simulink library "EmE_MBD_Blockset"  (R2018a)
settings: Solver=ode1  StartTime=0.0  StopTime=Inf  FixedStep=0.001  RelTol=1e-3  EnableMultiTasking=on
PostLoadFcn:
  | , if any(exist('dsrtsu_mdlpostloadfcn', 'file') == [2, 3, 6]), try dsrtsu_mdlpostloadfcn('Execute', bdroot); catch fprintf('Error in PostLoadFcn (dsrtsu_mdlpostloadfcn) for model "%s":\n %s\n', bdroot, lasterr); end, end,
undefined symbols (not defined in the file or in its folder): ENUM_TSC1_CONTROL_PURPOSE_T, gcbh, GLB_SWITCH_T
libraries: simulink x237, $bdroot x115, simulink_need_slupdate x26, MotoHawk_lib x13, simulink_extras x3
(part 5 of 11)

== system EmE_MBD_Blockset/Discrete/PT1_First_order_lag/Cubic_Approximation ==
  In1 : Inport
  Add2 : Sum  Inputs=++++  InputSameDT=on
  Constant2 : Constant
  Product{4..8} (5 alike) : Product  InputSameDT=on
  cubic_appr_x2_factor : Constant  Value=0.468222
  cubic_appr_x3_factor : Constant  Value=0.105562
  cubic_appr_x_factor : Constant  Value=0.995043
  Out1 : Outport
  wires:
  Product4/1 -> Product7/1, Product5/1
  cubic_appr_x_factor/1 -> Product6/2
  Product8/1 -> Add2/4
  cubic_appr_x3_factor/1 -> Product8/2
  Product5/1 -> Product8/1
  cubic_appr_x2_factor/1 -> Product7/2
  Product6/1 -> Add2/2
  Add2/1 -> Out1/1
  Product7/1 -> Add2/3
  Constant2/1 -> Add2/1
  In1/1 -> Product4/1, Product4/2, Product5/2, Product6/1

== system EmE_MBD_Blockset/Discrete/Turn_off_delay/SR flip-flop1 ==
  Sp : Inport
  R : Inport  Port=2
  Logical Operator : Logic  OutDataTypeStr=boolean
  Logical Operator1 : Logic  Operator=OR  OutDataTypeStr=boolean
  Logical Operator2 : Logic  Operator=NOT  OutDataTypeStr=boolean
  Logical Operator3 : Logic  Operator=NOT  OutDataTypeStr=boolean
  Unit_Delay : UnitDelay  InitialCondition=false  SampleTime=-1
      settings: AttributesFormatString=IC: %<vinit>
  Q : Outport
  !Q : Outport  Port=2
  wires:
  Logical Operator2/1 -> !Q/1
  Sp/1 -> Logical Operator1/1
  Logical Operator1/1 -> Q/1, Unit_Delay/1, Logical Operator2/1
  Logical Operator/1 -> Logical Operator1/2
  Logical Operator3/1 -> Logical Operator/1
  Unit_Delay/1 -> Logical Operator/2
  R/1 -> Logical Operator3/1

== system EmE_MBD_Blockset/Logic and Bit Operations/D flip-flop with SR/Enabled and Triggered Subsystem ==
  In1 : Inport  LatchByDelayingOutsideSignal=on
  Enable : EnablePort
  Trigger : TriggerPort  VariantControl=(inherit)  StatesWhenEnabling=reset
  Logical Operator : Logic  Operator=NOT  OutDataTypeStr=boolean
  Out1 : Outport  OutputWhenDisabled=reset  InitialOutput=false
  Out2 : Outport  Port=2  OutputWhenDisabled=reset  InitialOutput=true
  wires:
  In1/1 -> Logical Operator/1, Out1/1
  Logical Operator/1 -> Out2/1

== system EmE_MBD_Blockset/User-Defined Functions/Snoop/CCP_ETC_SS1 ==
  note: Define Signal information for desired signals
  note: Calculate and Track
      | current PID and Offset
  note: Detect if the new CCP command is
      | new and one of interest.
  note: Continuously decode all
      | CCP commands
  note: Form the message pairing
      | only after recieving a
      | WRITE_DAQ message
      | command
  function : TriggerPort  TriggerType=function-call  VariantControl=(inherit)
  Bus Selector : BusSelector  OutputSignals=ODT_Number,DAQ_Number
  Bus Selector1 : BusSelector  OutputSignals=Element_Size,Memory_Address
  CCP Signal Data Configuration : Subsystem
  Calculate Data Location : Subsystem
  Process CCP Commands : Subsystem
  Read CAN Raw1 : MotoHawk_lib/CAN Blocks/Read CAN Raw  nam='CAN_2'  bus=-2  id_ext=1  id=hex2dec('EF00F8')  id_mask=hex2dec('1fffffff')  pay=[]  pay_mask=[]  queue=20  slot='CCP_ATI'  valid=off  stale=on
      settings: SourceProductName=MotoHawk
  Recieve Count : Subsystem
      mask Display: disp('RCV COUNT')
  Signal Data Pairing : Subsystem
  Terminator{,1..3,5} (5 alike) : Terminator
  Update Detect : Subsystem
  DAQ_Info : Outport
  wires:
  Process CCP Commands/6(STRT_STP) -> Signal Data Pairing/5(STRT_STP)
  Bus Selector/2 -> Calculate Data Location/5(DAQ_Number)  "<DAQ_Number>"
  Read CAN Raw1/5 -> Process CCP Commands/1(CCP_Raw)
  Signal Data Pairing/1(DAQ_Info) -> DAQ_Info/1
  CCP Signal Data Configuration/1(CCP_Signal_Info) -> Signal Data Pairing/6(Signal_Info)
  Calculate Data Location/2(Offset) -> Signal Data Pairing/3(Offset)
  Calculate Data Location/1(PID) -> Signal Data Pairing/2(PID)
  Update Detect/2(Set_Update) -> Calculate Data Location/2(Set_Update)
  Update Detect/1(Write_Update) -> Signal Data Pairing/1(Write_Update), Calculate Data Location/1(Write_Update)
  Bus Selector1/1 -> Calculate Data Location/6(Element_Size)  "<Element_Size>"
  Bus Selector/1 -> Calculate Data Location/4(ODT_Number)  "<ODT_Number>"
  Process CCP Commands/3(GET) -> Terminator/1
  Bus Selector1/2 -> Signal Data Pairing/4(Memory_Address)  "<Memory_Address>"
  Process CCP Commands/5(WRITE) -> Bus Selector1/1
  Process CCP Commands/4(SET) -> Bus Selector/1
  Process CCP Commands/2(Newest_Cmd) -> Update Detect/2(Newest_Cmd), Calculate Data Location/3(Newest_CMD)
  Process CCP Commands/1(CTR) -> Update Detect/1(CTR)
  Read CAN Raw1/1 -> Terminator2/1
  Read CAN Raw1/4 -> Terminator1/1
  Read CAN Raw1/3 -> Terminator5/1
  Read CAN Raw1/2 -> Terminator3/1

== system EmE_MBD_Blockset/User-Defined Functions/Snoop/CCP_ETC_SS2 ==
  DAQ_Info : Inport
  function : TriggerPort  TriggerType=function-call  VariantControl=(inherit)
  CCP_Parameter_Decode : Subsystem
  Read CAN Raw : MotoHawk_lib/CAN Blocks/Read CAN Raw  nam='CAN_2'  bus=-2  id_ext=1  id=hex2dec('1CEFF800')  id_mask=hex2dec('1fffffff')  pay=[]  pay_mask=[]  queue=10  slot='CCP_ETC'  valid=off  stale=off
      settings: SourceProductName=MotoHawk
  Recieve Count : Subsystem
      mask Display: disp('RCV COUNT')
  Terminator1 : Terminator
  Terminator2 : Terminator
  Terminator4 : Terminator
  RCV_DATA : Outport
  wires:
  DAQ_Info/1 -> CCP_Parameter_Decode/1(DAQ_Info)
  Read CAN Raw/4 -> CCP_Parameter_Decode/2(Data)
  CCP_Parameter_Decode/1(CCP_Parameters) -> RCV_DATA/1
  Read CAN Raw/3 -> Terminator2/1
  Read CAN Raw/2 -> Terminator1/1
  Read CAN Raw/1 -> Terminator4/1

== system EmE_MBD_Blockset/User-Defined Functions/Snoop/Defaulting ==
  RCV_DATA : Inport
  DAQ_Info : Inport  Port=2
  function : TriggerPort  TriggerType=function-call  VariantControl=(inherit)
  Bus Creator : BusCreator  Inputs=24
  Bus Creator1 : BusCreator  Inputs=2
  Bus Selector3 : BusSelector  OutputSignals=Data.Signal1,Info.Signal_Def1.F_Defined,Data.Signal2,Info.Signal_Def2.F_Defined,Data.Signal3,Info.Signal_Def3.F_Defined,Data.Signal4,Info.Signal_Def4.F_Defined,Data.Signal5,Info.Signal_Def5.F_Defined,Data.Signal6,Info.Signal_Def6.F_Defined,Data.Signal7,Info.Signal_Def7.F_Defined,Data.Signal8,Info.Signal_Def8.F_Defined,Data.Signal9,Info.Signal_Def9.F_Defined,Data.Signal10,Info.Signal_Def10.F_Defined,Data.Signal11,Info.Signal_Def11.F_Defined,Data.Signal12,Info.Signal_Def12.F_Defined
  DEFAULT1 : Subsystem  mask{Parameter1=12}
      mask prompts: Parameter1 "CCP_SIG_DEFAULT"
      mask Display: disp(get(gcbh,'name'))
  DEFAULT10 : Subsystem  mask{Parameter1=12}
      mask prompts: Parameter1 "CCP_SIG_DEFAULT"
      mask Display: disp(get(gcbh,'name'))
  DEFAULT11 : Subsystem  mask{Parameter1=12}
      mask prompts: Parameter1 "CCP_SIG_DEFAULT"
      mask Display: disp(get(gcbh,'name'))
  DEFAULT12 : Subsystem  mask{Parameter1=12}
      mask prompts: Parameter1 "CCP_SIG_DEFAULT"
      mask Display: disp(get(gcbh,'name'))
  DEFAULT2 : Subsystem  mask{Parameter1=12}
      mask prompts: Parameter1 "CCP_SIG_DEFAULT"
      mask Display: disp(get(gcbh,'name'))
  DEFAULT3 : Subsystem  mask{Parameter1=12}
      mask prompts: Parameter1 "CCP_SIG_DEFAULT"
      mask Display: disp(get(gcbh,'name'))
  DEFAULT4 : Subsystem  mask{Parameter1=12}
      mask prompts: Parameter1 "CCP_SIG_DEFAULT"
      mask Display: disp(get(gcbh,'name'))
  DEFAULT5 : Subsystem  mask{Parameter1=12}
      mask prompts: Parameter1 "CCP_SIG_DEFAULT"
      mask Display: disp(get(gcbh,'name'))
  DEFAULT6 : Subsystem  mask{Parameter1=12}
      mask prompts: Parameter1 "CCP_SIG_DEFAULT"
      mask Display: disp(get(gcbh,'name'))
  DEFAULT7 : Subsystem  mask{Parameter1=12}
      mask prompts: Parameter1 "CCP_SIG_DEFAULT"
      mask Display: disp(get(gcbh,'name'))
  DEFAULT8 : Subsystem  mask{Parameter1=12}
      mask prompts: Parameter1 "CCP_SIG_DEFAULT"
      mask Display: disp(get(gcbh,'name'))
  DEFAULT9 : Subsystem  mask{Parameter1=12}
      mask prompts: Parameter1 "CCP_SIG_DEFAULT"
      mask Display: disp(get(gcbh,'name'))
  Recieve Count : Subsystem
      mask Display: disp('DFLT COUNT')
  motohawk_calibration2 : MotoHawk_lib/Calibration & Probing Blocks/motohawk_calibration  nam='CCP_SNOOP_RESET_DELAY'  val=100  storage=Calibration  show_more=on  name_source=Use Parameter  data_type=Inherit via back propagation  read_level=1  write_level=1  ovr_cals=on  view_as=Number  enum_struct={'Disabled', 'Enabled'}  vector_style=Wide Row  use_help_units=off  help=''  units=''  use_header_enum=off  row_header_enum={}  col_header_enum={}  use_min_max=off  min_val=-inf  max_val=inf  use_precision=off  precision=''  gain=1  offset=0  exp=1  use_mototune_group=on  mototune_group='CCP_Snoop'  data_stores=motohawk_sfun_calibration_data_stores
      settings: SourceProductName=MotoHawk
  CCP_ETC_Data : Outport
  wires:
  motohawk_calibration2/1 -> DEFAULT2/2(reset_delay), DEFAULT3/2(reset_delay), DEFAULT4/2(reset_delay), DEFAULT5/2(reset_delay), DEFAULT6/2(reset_delay), DEFAULT7/2(reset_delay), DEFAULT8/2(reset_delay), DEFAULT9/2(reset_delay), DEFAULT10/2(reset_delay), DEFAULT11/2(reset_delay), DEFAULT12/2(reset_delay), DEFAULT1/2(reset_delay)
  Bus Creator/1 -> CCP_ETC_Data/1
  DEFAULT12/2(F_Defined) -> Bus Creator/24  "CA_Vehicle_speed_defined"
  DEFAULT12/1(Signal) -> Bus Creator/23  "CA_Vehicle_speed"
  DEFAULT11/2(F_Defined) -> Bus Creator/22  "CPM_Crank_power_defined"
  DEFAULT11/1(Signal) -> Bus Creator/21  "CPM_Crank_power"
  DEFAULT10/2(F_Defined) -> Bus Creator/20  "Air_temp_post_int_Value_defined"
  DEFAULT10/1(Signal) -> Bus Creator/19  "Air_temp_post_int_Value"
  DEFAULT9/2(F_Defined) -> Bus Creator/18  "F_CPM_Int_enabled_defined"
  DEFAULT9/1(Signal) -> Bus Creator/17  "F_CPM_Int_enabled"
  DEFAULT8/2(F_Defined) -> Bus Creator/16  "CREC_Eng_run_time_since_key_on_defined"
  DEFAULT8/1(Signal) -> Bus Creator/15  "CREC_Eng_run_time_since_key_on"
  DEFAULT7/2(F_Defined) -> Bus Creator/14  "CA_Cool_temp_value_defined"
  DEFAULT7/1(Signal) -> Bus Creator/13  "CA_Cool_temp_value"
  DEFAULT6/2(F_Defined) -> Bus Creator/12  "CA_Engine_speed_defined"
  DEFAULT6/1(Signal) -> Bus Creator/11  "CA_Engine_speed"
  DEFAULT5/2(F_Defined) -> Bus Creator/10  "CA_Ambient_air_press_value_defined"
  DEFAULT5/1(Signal) -> Bus Creator/9  "CA_Ambient_air_press_value"
  DEFAULT4/2(F_Defined) -> Bus Creator/8  "AMF_Fresh_air_defined"
  DEFAULT4/1(Signal) -> Bus Creator/7  "AMF_Fresh_air"
  DEFAULT3/2(F_Defined) -> Bus Creator/6  "CPM_Air_temp_pre_int_defined"
  DEFAULT3/1(Signal) -> Bus Creator/5  "CPM_Air_temp_pre_int"
  DEFAULT2/2(F_Defined) -> Bus Creator/4  "CA_Ecfan_fspd_value_defined"
  DEFAULT2/1(Signal) -> Bus Creator/3  "CA_Ecfan_fspd_value"
  Bus Selector3/24 -> DEFAULT12/3(f_defined)  "<F_Defined>"
  Bus Selector3/23 -> DEFAULT12/1(signal)  "<Signal12>"
  Bus Selector3/22 -> DEFAULT11/3(f_defined)  "<F_Defined>"
  Bus Selector3/21 -> DEFAULT11/1(signal)  "<Signal11>"
  Bus Selector3/20 -> DEFAULT10/3(f_defined)  "<F_Defined>"
  Bus Selector3/19 -> DEFAULT10/1(signal)  "<Signal10>"
  Bus Selector3/18 -> DEFAULT9/3(f_defined)  "<F_Defined>"
  Bus Selector3/17 -> DEFAULT9/1(signal)  "<Signal9>"
  Bus Selector3/16 -> DEFAULT8/3(f_defined)  "<F_Defined>"
  Bus Selector3/15 -> DEFAULT8/1(signal)  "<Signal8>"
  Bus Selector3/14 -> DEFAULT7/3(f_defined)  "<F_Defined>"
  Bus Selector3/13 -> DEFAULT7/1(signal)  "<Signal7>"
  Bus Selector3/12 -> DEFAULT6/3(f_defined)  "<F_Defined>"
  Bus Selector3/11 -> DEFAULT6/1(signal)  "<Signal6>"
  Bus Selector3/10 -> DEFAULT5/3(f_defined)  "<F_Defined>"
  Bus Selector3/9 -> DEFAULT5/1(signal)  "<Signal5>"
  Bus Selector3/8 -> DEFAULT4/3(f_defined)  "<F_Defined>"
  Bus Selector3/7 -> DEFAULT4/1(signal)  "<Signal4>"
  Bus Selector3/6 -> DEFAULT3/3(f_defined)  "<F_Defined>"
  Bus Selector3/5 -> DEFAULT3/1(signal)  "<Signal3>"
  Bus Selector3/4 -> DEFAULT2/3(f_defined)  "<F_Defined>"
  Bus Selector3/3 -> DEFAULT2/1(signal)  "<Signal2>"
  Bus Selector3/2 -> DEFAULT1/3(f_defined)  "<F_Defined>"
  Bus Selector3/1 -> DEFAULT1/1(signal)  "<Signal1>"
  RCV_DATA/1 -> Bus Creator1/1  "Data"
  Bus Creator1/1 -> Bus Selector3/1
  DEFAULT1/2(F_Defined) -> Bus Creator/2  "CA_Ambient_air_temp_value_defined"
  DEFAULT1/1(Signal) -> Bus Creator/1  "CA_Ambient_air_temp_value"
  DAQ_Info/1 -> Bus Creator1/2  "Info"

== system EmE_MBD_Blockset/Controllers/Generic_PID_Governor_3/Calculate_PID_terms/Calculate_D_term ==
  GPID_Kd : Inport
  GPID_dT : Inport  Port=2
  F_GPID_reset_gov : Inport  Port=3
  GPID_control_error : Inport  Port=4
  GPID_T_filt_d : Inport  Port=5
  Enable : EnablePort  StatesWhenEnabling=reset
      settings: AttributesFormatString=States when enabling: %<StatesWhenEnabling>
  Divide : Product  Inputs=*/*  InputSameDT=on
  LPF_first_order : $bdroot/Discrete/LPF_first_order
  Subtract : Sum  Inputs=+-  InputSameDT=on
  Unit Delay Resettable External IC : simulink_need_slupdate/Unit Delay Resettable External IC  tsamp=-1
      settings: SourceProductName=Simulink  SourceProductBaseCode=SL
  GPID_d_term : Outport  OutputWhenDisabled=reset  InitialOutput=0
      settings: AttributesFormatString=IC: %<InitialOutput>\nDisabled value: %<OutputWhenDisabled>
  wires:
  GPID_control_error/1 -> LPF_first_order/2, LPF_first_order/3
  F_GPID_reset_gov/1 -> Unit Delay Resettable External IC/2, LPF_first_order/1
  GPID_dT/1 -> Divide/2, LPF_first_order/5
  GPID_T_filt_d/1 -> LPF_first_order/4
  LPF_first_order/1 -> Divide/1
  GPID_Kd/1 -> Divide/3
  Divide/1 -> Subtract/1, Unit Delay Resettable External IC/1, Unit Delay Resettable External IC/3
  Unit Delay Resettable External IC/1 -> Subtract/2
  Subtract/1 -> GPID_d_term/1

== system EmE_MBD_Blockset/Controllers/Generic_PID_Governor_3/Calculate_PID_terms/Calculate_I_term ==
  GPID_p_term : Inport
  GPID_Ki : Inport  Port=2
  GPID_actual_system_output : Inport  Port=3
  GPID_control_error : Inport  Port=4
  F_GPID_reset_gov : Inport  Port=5
  GPID_dT : Inport  Port=6
  GPID_feed_forward : Inport  Port=7
  F_GPID_aw_cond_integration : Inport  Port=8
  GPID_aw_hysteresis : Inport  Port=9
  F_GPID_aw_hold_i_term : Inport  Port=10
  GPID_output_unlim_prev : Inport  Port=11
  Enable : EnablePort  StatesWhenEnabling=reset
      settings: AttributesFormatString=States when enabling: %<StatesWhenEnabling>
  Calculate_integral_term : Subsystem
  Initialize_integral_term : Subsystem
  Prevent_integral_term_windup : Subsystem
  Unit_Delay : UnitDelay  SampleTime=-1
      settings: AttributesFormatString=IC: %<vinit>
  GPID_i_term : Outport  OutputWhenDisabled=reset  InitialOutput=0
      settings: AttributesFormatString=IC: %<InitialOutput>\nDisabled value: %<OutputWhenDisabled>
  F_GPID_hold_i_term : Outport  Port=2  OutputWhenDisabled=reset  InitialOutput=false
      settings: AttributesFormatString=IC: %<InitialOutput>\nDisabled value: %<OutputWhenDisabled>
  wires:
  Calculate_integral_term/1(GPID_i_term) -> GPID_i_term/1, Unit_Delay/1
  Initialize_integral_term/1(GPID_i_sum_error_init) -> Calculate_integral_term/3(GPID_i_sum_error_init)
  Prevent_integral_term_windup/1(F_GPID_hold_i_term) -> Calculate_integral_term/6(F_GPID_hold_i_term), F_GPID_hold_i_term/1
  GPID_dT/1 -> Initialize_integral_term/1(GPID_dT), Calculate_integral_term/1(GPID_dT)
  F_GPID_reset_gov/1 -> Prevent_integral_term_windup/4(F_GPID_reset_gov), Initialize_integral_term/Enable, Calculate_integral_term/2(F_GPID_reset_gov)
  GPID_feed_forward/1 -> Initialize_integral_term/2(GPID_feed_forward)
  GPID_Ki/1 -> Initialize_integral_term/6(GPID_Ki), Calculate_integral_term/5(GPID_Ki), Prevent_integral_term_windup/1(GPID_Ki)
  GPID_control_error/1 -> Initialize_integral_term/5(GPID_control_error), Calculate_integral_term/4(GPID_control_error), Prevent_integral_term_windup/2(GPID_control_error)
  GPID_actual_system_output/1 -> Initialize_integral_term/4(GPID_actual_system_output), Prevent_integral_term_windup/3(GPID_actual_system_output)
  GPID_p_term/1 -> Initialize_integral_term/3(GPID_p_term)
  GPID_output_unlim_prev/1 -> Prevent_integral_term_windup/5(GPID_output_unlim_prev)
  F_GPID_aw_cond_integration/1 -> Prevent_integral_term_windup/6(F_GPID_aw_cond_integration)
  GPID_aw_hysteresis/1 -> Prevent_integral_term_windup/7(GPID_aw_hysteresis)
  F_GPID_aw_hold_i_term/1 -> Prevent_integral_term_windup/8(F_GPID_aw_hold_i_term)
  Unit_Delay/1 -> Prevent_integral_term_windup/9(GPID_i_term_prev)

== system EmE_MBD_Blockset/Controllers/Generic_PID_Governor_3/Calculate_PID_terms/Calculate_P_term ==
  GPID_Kp : Inport
  GPID_control_error : Inport  Port=2
  Product : Product  InputSameDT=on
  GPID_p_term : Outport
  wires:
  Product/1 -> GPID_p_term/1
  GPID_control_error/1 -> Product/2
  GPID_Kp/1 -> Product/1

== system EmE_MBD_Blockset/Controllers/Generic_PID_Governor_4/Calculate_PID_terms/Calculate_D_term ==
  GPID_Kd : Inport
  GPID_dT : Inport  Port=2
  F_GPID_reset_gov : Inport  Port=3
  GPID_control_error : Inport  Port=4
  GPID_T_filt_d : Inport  Port=5
  Enable : EnablePort  StatesWhenEnabling=reset
      settings: AttributesFormatString=States when enabling: %<StatesWhenEnabling>
  Divide : Product  Inputs=*/*  InputSameDT=on
  LPF_first_order : $bdroot/Discrete/LPF_first_order
  Subtract : Sum  Inputs=+-  InputSameDT=on
  Unit Delay Resettable External IC : simulink_need_slupdate/Unit Delay Resettable External IC  tsamp=-1
      settings: SourceProductName=Simulink  SourceProductBaseCode=SL
  GPID_d_term : Outport  OutputWhenDisabled=reset  InitialOutput=0
      settings: AttributesFormatString=IC: %<InitialOutput>\nDisabled value: %<OutputWhenDisabled>
  wires:
  GPID_control_error/1 -> LPF_first_order/2, LPF_first_order/3
  F_GPID_reset_gov/1 -> Unit Delay Resettable External IC/2, LPF_first_order/1
  GPID_dT/1 -> Divide/2, LPF_first_order/5
  GPID_T_filt_d/1 -> LPF_first_order/4
  LPF_first_order/1 -> Divide/1
  GPID_Kd/1 -> Divide/3
  Divide/1 -> Subtract/1, Unit Delay Resettable External IC/1, Unit Delay Resettable External IC/3
  Unit Delay Resettable External IC/1 -> Subtract/2
  Subtract/1 -> GPID_d_term/1

== system EmE_MBD_Blockset/Controllers/Generic_PID_Governor_4/Calculate_PID_terms/Calculate_I_term ==
  GPID_p_term : Inport
  GPID_Ki : Inport  Port=2
  GPID_actual_system_output : Inport  Port=3
  GPID_control_error : Inport  Port=4
  F_GPID_reset_gov : Inport  Port=5
  GPID_dT : Inport  Port=6
  GPID_feed_forward : Inport  Port=7
  F_GPID_aw_cond_integration : Inport  Port=8
  GPID_aw_hysteresis : Inport  Port=9
  F_GPID_aw_hold_i_term : Inport  Port=10
  GPID_output_unlim_prev : Inport  Port=11
  GPID_output_delta : Inport  Port=12
  Enable : EnablePort  StatesWhenEnabling=reset
      settings: AttributesFormatString=States when enabling: %<StatesWhenEnabling>
  Calculate_integral_term : Subsystem
  Initialize_integral_term : Subsystem
  Prevent_integral_term_windup : Subsystem
  Unit_Delay : UnitDelay  SampleTime=-1
      settings: AttributesFormatString=IC: %<vinit>
  GPID_i_term : Outport  OutputWhenDisabled=reset  InitialOutput=0
      settings: AttributesFormatString=IC: %<InitialOutput>\nDisabled value: %<OutputWhenDisabled>
  F_GPID_hold_i_term : Outport  Port=2  OutputWhenDisabled=reset  InitialOutput=false
      settings: AttributesFormatString=IC: %<InitialOutput>\nDisabled value: %<OutputWhenDisabled>
  wires:
  Calculate_integral_term/1(GPID_i_term) -> GPID_i_term/1, Unit_Delay/1
  Initialize_integral_term/1(GPID_i_sum_error_init) -> Calculate_integral_term/3(GPID_i_sum_error_init)
  Prevent_integral_term_windup/1(F_GPID_hold_i_term) -> Calculate_integral_term/7(F_GPID_hold_i_term), F_GPID_hold_i_term/1
  GPID_dT/1 -> Initialize_integral_term/1(GPID_dT), Calculate_integral_term/1(GPID_dT)
  F_GPID_reset_gov/1 -> Prevent_integral_term_windup/4(F_GPID_reset_gov), Initialize_integral_term/Enable, Calculate_integral_term/2(F_GPID_reset_gov)
  GPID_feed_forward/1 -> Initialize_integral_term/2(GPID_feed_forward)
  GPID_Ki/1 -> Initialize_integral_term/6(GPID_Ki), Calculate_integral_term/5(GPID_Ki), Prevent_integral_term_windup/1(GPID_Ki)
  GPID_control_error/1 -> Initialize_integral_term/5(GPID_control_error), Calculate_integral_term/4(GPID_control_error), Prevent_integral_term_windup/2(GPID_control_error)
  GPID_actual_system_output/1 -> Initialize_integral_term/4(GPID_actual_system_output), Prevent_integral_term_windup/3(GPID_actual_system_output)
  GPID_p_term/1 -> Initialize_integral_term/3(GPID_p_term)
  GPID_output_unlim_prev/1 -> Prevent_integral_term_windup/5(GPID_output_unlim_prev)
  F_GPID_aw_cond_integration/1 -> Prevent_integral_term_windup/6(F_GPID_aw_cond_integration)
  GPID_aw_hysteresis/1 -> Prevent_integral_term_windup/7(GPID_aw_hysteresis)
  F_GPID_aw_hold_i_term/1 -> Prevent_integral_term_windup/8(F_GPID_aw_hold_i_term)
  Unit_Delay/1 -> Prevent_integral_term_windup/9(GPID_i_term_prev)
  GPID_output_delta/1 -> Calculate_integral_term/6(GPID_output_delta)

== system EmE_MBD_Blockset/Controllers/Generic_PID_Governor_4/Calculate_PID_terms/Calculate_P_term ==
  GPID_Kp : Inport
  GPID_control_error : Inport  Port=2
  Product : Product  InputSameDT=on
  GPID_p_term : Outport
  wires:
  Product/1 -> GPID_p_term/1
  GPID_control_error/1 -> Product/2
  GPID_Kp/1 -> Product/1

== system EmE_MBD_Blockset/User-Defined Functions/Snoop/CCP_ETC_SS1/CCP Signal Data Configuration ==
  note: Use Byte 1
      | 0 = Float
      | 1 = Use
  note: Use Byte 2
      | 0 = Don't Use
      | 1 = Use
  note: Use Byte 3-4
      | 0 = Don't Use
      | 1 = Use
  note: Signage
      | 0 = Unsigned
      | 1 = Signed
  note: Signal Types
      | 0001 = uchar     UBYTE                    1   BYTE         unsigned 8 Bit
      | 1001 = char       SBYTE                    1   char            signed 8 Bit
      | 0011 = uint        UWORD                   2   WORD        unsigned integer 16 Bit
      | 1011 = int          SWORD                   2   int              signed integer 16 Bit
      | 0111 = ulong     ULONG                   4    DWORD     unsigned integer 32 Bit
      | 1111 = long       SLONG                   4    LONG        signed integer 32 Bit
      | 0000 = float       FLOAT32_IEEE      4                     float 32 Bit
  Bus Creator1 : BusCreator  Inputs=12
  FLOAT32 : Constant  Value=bin2dec('0000')  OutDataTypeStr=uint8
  SBYTE : Constant  Value=bin2dec('1001')  OutDataTypeStr=uint8
  SLONG : Constant  Value=bin2dec('1111')  OutDataTypeStr=uint8
  SWORD : Constant  Value=bin2dec('1011')  OutDataTypeStr=uint8
  SignalDef1 : Subsystem  mask(SignalDef){sigName=CA_Ambient_air_temp_value, address=400076EC, sigType=single, sigConvert=[1  1  0], sigDefault=0}
      mask prompts: sigName "Signal Name"; address "Signal A2L Address"; sigType "Signal Type"; sigConvert "Signal conversion vector [A B C] :: (A/B) * x + C"; sigDefault "Default Value"
      mask init:
      | signal_def_init;
      mask TypeOptions sigType: uint8 | int8 | uint16 | int16 | uint32 | int32 | single
      mask Display:
      | text(.5,.5, sigName, 'HorizontalAlign', 'Center')
      | patch([0.1 0.9 0.9 0.1], [0.15 0.15 0.10 0.10], [1 1 1])
  SignalDef10 : Subsystem  mask(SignalDef){sigName=Air_temp_post_int_Value, address=00501F12, sigType=uint16, sigConvert=[1  10   0], sigDefault=0}
      mask prompts: sigName "Signal Name"; address "Signal A2L Address"; sigType "Signal Type"; sigConvert "Signal conversion vector [A B C] :: (A/B) * x + C"; sigDefault "Default Value"
      mask init:
      | signal_def_init;
      mask TypeOptions sigType: uint8 | int8 | uint16 | int16 | uint32 | int32 | single
      mask Display:
      | text(.5,.5, sigName, 'HorizontalAlign', 'Center')
      | patch([0.1 0.9 0.9 0.1], [0.15 0.15 0.10 0.10], [1 1 1])
  SignalDef11 : Subsystem  mask(SignalDef){sigName=CPM_Crank_power, address=4000C33C, sigType=int16, sigConvert=[1  10   0], sigDefault=0}
      mask prompts: sigName "Signal Name"; address "Signal A2L Address"; sigType "Signal Type"; sigConvert "Signal conversion vector [A B C] :: (A/B) * x + C"; sigDefault "Default Value"
      mask init:
      | signal_def_init;
      mask TypeOptions sigType: uint8 | int8 | uint16 | int16 | uint32 | int32 | single
      mask Display:
      | text(.5,.5, sigName, 'HorizontalAlign', 'Center')
      | patch([0.1 0.9 0.9 0.1], [0.15 0.15 0.10 0.10], [1 1 1])
  SignalDef12 : Subsystem  mask(SignalDef){sigName=CA_Vehicle_speed, address=40007564, sigType=single, sigConvert=[1  1  0], sigDefault=0}
      mask prompts: sigName "Signal Name"; address "Signal A2L Address"; sigType "Signal Type"; sigConvert "Signal conversion vector [A B C] :: (A/B) * x + C"; sigDefault "Default Value"
      mask init:
      | signal_def_init;
      mask TypeOptions sigType: uint8 | int8 | uint16 | int16 | uint32 | int32 | single
      mask Display:
      | text(.5,.5, sigName, 'HorizontalAlign', 'Center')
      | patch([0.1 0.9 0.9 0.1], [0.15 0.15 0.10 0.10], [1 1 1])
  SignalDef2 : Subsystem  mask(SignalDef){sigName=CA_Ecfan_fspd_value, address=40007D66, sigType=uint16, sigConvert=[1  1  0], sigDefault=0}
      mask prompts: sigName "Signal Name"; address "Signal A2L Address"; sigType "Signal Type"; sigConvert "Signal conversion vector [A B C] :: (A/B) * x + C"; sigDefault "Default Value"
      mask init:
      | signal_def_init;
      mask TypeOptions sigType: uint8 | int8 | uint16 | int16 | uint32 | int32 | single
      mask Display:
      | text(.5,.5, sigName, 'HorizontalAlign', 'Center')
      | patch([0.1 0.9 0.9 0.1], [0.15 0.15 0.10 0.10], [1 1 1])
  SignalDef3 : Subsystem  mask(SignalDef){sigName=CPM_Air_temp_pre_int, address=4000C33A, sigType=uint16, sigConvert=[1  10   0], sigDefault=0}
      mask prompts: sigName "Signal Name"; address "Signal A2L Address"; sigType "Signal Type"; sigConvert "Signal conversion vector [A B C] :: (A/B) * x + C"; sigDefault "Default Value"
      mask init:
      | signal_def_init;
      mask TypeOptions sigType: uint8 | int8 | uint16 | int16 | uint32 | int32 | single
      mask Display:
      | text(.5,.5, sigName, 'HorizontalAlign', 'Center')
      | patch([0.1 0.9 0.9 0.1], [0.15 0.15 0.10 0.10], [1 1 1])
  SignalDef4 : Subsystem  mask(SignalDef){sigName=AMF_Fresh_air, address=4000BF4A, sigType=uint16, sigConvert=[1  40   0], sigDefault=0}
      mask prompts: sigName "Signal Name"; address "Signal A2L Address"; sigType "Signal Type"; sigConvert "Signal conversion vector [A B C] :: (A/B) * x + C"; sigDefault "Default Value"
      mask init:
      | signal_def_init;
      mask TypeOptions sigType: uint8 | int8 | uint16 | int16 | uint32 | int32 | single
      mask Display:
      | text(.5,.5, sigName, 'HorizontalAlign', 'Center')
      | patch([0.1 0.9 0.9 0.1], [0.15 0.15 0.10 0.10], [1 1 1])
  SignalDef5 : Subsystem  mask(SignalDef){sigName=CA_Ambient_air_press_value, address=4000768C, sigType=single, sigConvert=[1  1  0], sigDefault=0}
      mask prompts: sigName "Signal Name"; address "Signal A2L Address"; sigType "Signal Type"; sigConvert "Signal conversion vector [A B C] :: (A/B) * x + C"; sigDefault "Default Value"
      mask init:
      | signal_def_init;
      mask TypeOptions sigType: uint8 | int8 | uint16 | int16 | uint32 | int32 | single
      mask Display:
      | text(.5,.5, sigName, 'HorizontalAlign', 'Center')
      | patch([0.1 0.9 0.9 0.1], [0.15 0.15 0.10 0.10], [1 1 1])
  SignalDef6 : Subsystem  mask(SignalDef){sigName=CA_Engine_speed, address=40007530, sigType=single, sigConvert=[1  1  0], sigDefault=0}
      mask prompts: sigName "Signal Name"; address "Signal A2L Address"; sigType "Signal Type"; sigConvert "Signal conversion vector [A B C] :: (A/B) * x + C"; sigDefault "Default Value"
      mask init:
      | signal_def_init;
      mask TypeOptions sigType: uint8 | int8 | uint16 | int16 | uint32 | int32 | single
      mask Display:
      | text(.5,.5, sigName, 'HorizontalAlign', 'Center')
      | patch([0.1 0.9 0.9 0.1], [0.15 0.15 0.10 0.10], [1 1 1])
  SignalDef7 : Subsystem  mask(SignalDef){sigName=CA_Cool_temp_value, address=4000750C, sigType=single, sigConvert=[1  1  0], sigDefault=0}
      mask prompts: sigName "Signal Name"; address "Signal A2L Address"; sigType "Signal Type"; sigConvert "Signal conversion vector [A B C] :: (A/B) * x + C"; sigDefault "Default Value"
      mask init:
      | signal_def_init;
      mask TypeOptions sigType: uint8 | int8 | uint16 | int16 | uint32 | int32 | single
      mask Display:
      | text(.5,.5, sigName, 'HorizontalAlign', 'Center')
      | patch([0.1 0.9 0.9 0.1], [0.15 0.15 0.10 0.10], [1 1 1])
  SignalDef8 : Subsystem  mask(SignalDef){sigName=CREC_Eng_run_time_since_key_on, address=40006210, sigType=uint32, sigConvert=[1  1  0], sigDefault=0}
      mask prompts: sigName "Signal Name"; address "Signal A2L Address"; sigType "Signal Type"; sigConvert "Signal conversion vector [A B C] :: (A/B) * x + C"; sigDefault "Default Value"
      mask init:
      | signal_def_init;
      mask TypeOptions sigType: uint8 | int8 | uint16 | int16 | uint32 | int32 | single
      mask Display:
      | text(.5,.5, sigName, 'HorizontalAlign', 'Center')
      | patch([0.1 0.9 0.9 0.1], [0.15 0.15 0.10 0.10], [1 1 1])
  SignalDef9 : Subsystem  mask(SignalDef){sigName=F_CPM_Int_enabled, address=4000C324, sigType=uint8, sigConvert=[1  1  0], sigDefault=0}
      mask prompts: sigName "Signal Name"; address "Signal A2L Address"; sigType "Signal Type"; sigConvert "Signal conversion vector [A B C] :: (A/B) * x + C"; sigDefault "Default Value"
      mask init:
      | signal_def_init;
      mask TypeOptions sigType: uint8 | int8 | uint16 | int16 | uint32 | int32 | single
      mask Display:
      | text(.5,.5, sigName, 'HorizontalAlign', 'Center')
      | patch([0.1 0.9 0.9 0.1], [0.15 0.15 0.10 0.10], [1 1 1])
  Terminator{,1..6} (7 alike) : Terminator
  UBYTE : Constant  Value=bin2dec('0001')  OutDataTypeStr=uint8
  ULONG : Constant  Value=bin2dec('0111')  OutDataTypeStr=uint8
  UWORD : Constant  Value=bin2dec('0011')  OutDataTypeStr=uint8
  CCP_Signal_Info : Outport
  wires:
  SignalDef12/1(Signal_Info) -> Bus Creator1/12  "Signal_Info12"
  SignalDef11/1(Signal_Info) -> Bus Creator1/11  "Signal_Info11"
  SignalDef10/1(Signal_Info) -> Bus Creator1/10  "Signal_Info10"
  SignalDef9/1(Signal_Info) -> Bus Creator1/9  "Signal_Info9"
  SignalDef8/1(Signal_Info) -> Bus Creator1/8  "Signal_Info8"
  SignalDef7/1(Signal_Info) -> Bus Creator1/7  "Signal_Info7"
  SignalDef6/1(Signal_Info) -> Bus Creator1/6  "Signal_Info6"
  UBYTE/1 -> Terminator/1
  SBYTE/1 -> Terminator1/1
  UWORD/1 -> Terminator2/1
  SWORD/1 -> Terminator3/1
  ULONG/1 -> Terminator4/1
  SLONG/1 -> Terminator5/1
  FLOAT32/1 -> Terminator6/1
  SignalDef5/1(Signal_Info) -> Bus Creator1/5  "Signal_Info5"
  SignalDef4/1(Signal_Info) -> Bus Creator1/4  "Signal_Info4"
  SignalDef3/1(Signal_Info) -> Bus Creator1/3  "Signal_Info3"
  SignalDef2/1(Signal_Info) -> Bus Creator1/2  "Signal_Info2"
  Bus Creator1/1 -> CCP_Signal_Info/1  "CCP_Signal_Info"
  SignalDef1/1(Signal_Info) -> Bus Creator1/1  "Signal_Info1"

== system EmE_MBD_Blockset/User-Defined Functions/Snoop/CCP_ETC_SS1/Calculate Data Location ==
  note: Increment only when element size is provided by a
      | WRITE_DAQ. The Element_Size signal will be meaningless
      | (but still calculated) when any other CCP command is recieved.
  note: Byte offset represents the signal's position within an ODT.
      | Each ODT contains up to 7 bytes of information (bytes 2-8).
      | Offest is Zero-indexed
  note: Counter for Byte Offset must reset whenever
      | a new ODT is used
  note: Actual PID is offset by ODT_number
      | from the first PID
  note: First PID Calibratible
      | - replace later with info from GET_DAQ
  Write_Update : Inport
  Set_Update : Inport  Port=2
  Newest_CMD : Inport  Port=3
  ODT_Number : Inport  Port=4
  DAQ_Number : Inport  Port=5
  Element_Size : Inport  Port=6
  Add : Sum  Inputs=+++  OutDataTypeStr=uint8
  Add1 : Sum
  CCP_SNOOP_DAQSIZE : Constant  Value=16  OutDataTypeStr=uint8
  CCP_SNOOP_FIRSTPID : Constant  Value=64  OutDataTypeStr=uint8
  Constant : Constant  Value=0  OutDataTypeStr=uint8
  Constant1 : Constant  Value=0  OutDataTypeStr=uint8
  GET_DAQ : Constant  Value=hex2dec('14')  OutDataTypeStr=uint8
  Logical Operator : Logic  Operator=OR  Inputs=3  AllPortsSameDT=off  OutDataTypeStr=boolean
  Product : Product  RndMeth=Zero
  Relational Operator : RelationalOperator  Operator=~=  OutDataTypeStr=boolean  RndMeth=Nearest
  Relational Operator1 : RelationalOperator  Operator===  OutDataTypeStr=boolean  RndMeth=Nearest
  Relational Operator2 : RelationalOperator  Operator=~=  OutDataTypeStr=boolean  RndMeth=Nearest
  Switch : Switch  Criteria=u2 ~= 0
  Switch1 : Switch  Criteria=u2 ~= 0
  Switch2 : Switch  Criteria=u2 ~= 0
  Unit Delay{1..4} (4 alike) : UnitDelay  SampleTime=-1
  PID : Outport
  Offset : Outport  Port=2
  wires:
  Write_Update/1 -> Switch1/2
  DAQ_Number/1 -> Relational Operator2/2, Product/1, Unit Delay4/1
  CCP_SNOOP_DAQSIZE/1 -> Product/2
  CCP_SNOOP_FIRSTPID/1 -> Add/2
  [F_NewDAQ] -> Logical Operator/3
  Relational Operator2/1 -> [F_NewDAQ]
  Unit Delay4/1 -> Relational Operator2/1
  Product/1 -> Add/1
  Newest_CMD/1 -> Relational Operator1/2
  Relational Operator1/1 -> Logical Operator/2
  Relational Operator/1 -> Logical Operator/1
  Logical Operator/1 -> Switch2/2
  GET_DAQ/1 -> Relational Operator1/1
  Unit Delay3/1 -> Add1/1
  Element_Size/1 -> Switch1/1
  ODT_Number/1 -> Switch/1
  Add/1 -> PID/1  "PID"
  Switch1/1 -> Unit Delay3/1
  Constant1/1 -> Switch1/3
  Unit Delay2/1 -> Add1/2
  Add1/1 -> Switch2/3
  Switch/1 -> Add/3, Relational Operator/1, Unit Delay1/1
  Set_Update/1 -> Switch/2
  Constant/1 -> Switch2/1
  Switch2/1 -> Offset/1, Unit Delay2/1  "current_elm_offset"
  Unit Delay1/1 -> Switch/3, Relational Operator/2

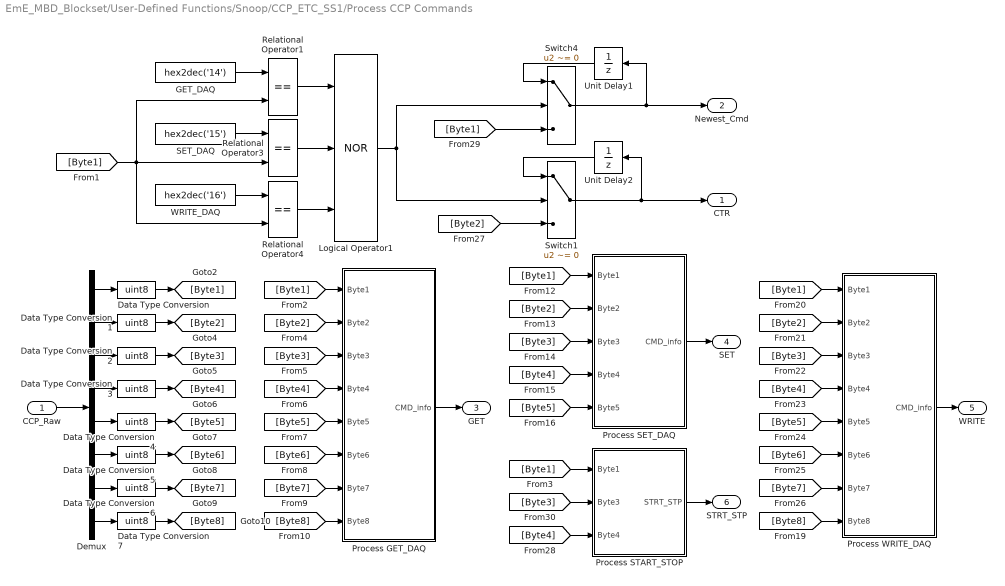
== system EmE_MBD_Blockset/User-Defined Functions/Snoop/CCP_ETC_SS1/Process CCP Commands ==
  CCP_Raw : Inport
  Data Type Conversion{,1..7} (8 alike) : DataTypeConversion  OutDataTypeStr=uint8
  Demux : Demux  Outputs=8
  GET_DAQ : Constant  Value=hex2dec('14')  OutDataTypeStr=uint8
  Logical Operator1 : Logic  Operator=NOR  Inputs=3  AllPortsSameDT=off  OutDataTypeStr=boolean
  Process GET_DAQ : Subsystem
  Process SET_DAQ : Subsystem
  Process START_STOP : Subsystem
  Process WRITE_DAQ : Subsystem
  Relational Operator1 : RelationalOperator  Operator===  OutDataTypeStr=boolean  RndMeth=Nearest
  Relational Operator3 : RelationalOperator  Operator===  OutDataTypeStr=boolean  RndMeth=Nearest
  Relational Operator4 : RelationalOperator  Operator===  OutDataTypeStr=boolean  RndMeth=Nearest
  SET_DAQ : Constant  Value=hex2dec('15')  OutDataTypeStr=uint8
  Switch1 : Switch  Criteria=u2 ~= 0
  Switch4 : Switch  Criteria=u2 ~= 0
  Unit Delay1 : UnitDelay  SampleTime=-1
  Unit Delay2 : UnitDelay  SampleTime=-1
  WRITE_DAQ : Constant  Value=hex2dec('16')  OutDataTypeStr=uint8
  CTR : Outport
  Newest_Cmd : Outport  Port=2
  GET : Outport  Port=3
  SET : Outport  Port=4
  WRITE : Outport  Port=5
  STRT_STP : Outport  Port=6
  wires:
  Relational Operator1/1 -> Logical Operator1/1
  Relational Operator3/1 -> Logical Operator1/2
  Relational Operator4/1 -> Logical Operator1/3
  [Byte3] -> Process START_STOP/2(Byte3)
  [Byte4] -> Process START_STOP/3(Byte4)
  [Byte1] -> Process START_STOP/1(Byte1)
  Process START_STOP/1(STRT_STP) -> STRT_STP/1
  [Byte2] -> Switch1/3
  Unit Delay2/1 -> Switch1/1
  Switch1/1 -> Unit Delay2/1, CTR/1
  [Byte1] -> Process SET_DAQ/1(Byte1)
  [Byte2] -> Process SET_DAQ/2(Byte2)
  [Byte3] -> Process SET_DAQ/3(Byte3)
  [Byte4] -> Process SET_DAQ/4(Byte4)
  [Byte5] -> Process SET_DAQ/5(Byte5)
  Unit Delay1/1 -> Switch4/1
  Switch4/1 -> Newest_Cmd/1, Unit Delay1/1
  [Byte1] -> Switch4/3
  Demux/1 -> Data Type Conversion/1
  Demux/2 -> Data Type Conversion1/1
  Demux/3 -> Data Type Conversion2/1
  Demux/4 -> Data Type Conversion3/1
  Demux/5 -> Data Type Conversion4/1
  Demux/6 -> Data Type Conversion5/1
  Demux/7 -> Data Type Conversion6/1
  Demux/8 -> Data Type Conversion7/1
  Data Type Conversion1/1 -> [Byte2]
  Data Type Conversion3/1 -> [Byte4]
  Data Type Conversion4/1 -> [Byte5]
  Data Type Conversion6/1 -> [Byte7]
  Data Type Conversion7/1 -> [Byte8]
  Data Type Conversion/1 -> [Byte1]
  Data Type Conversion2/1 -> [Byte3]
  Data Type Conversion5/1 -> [Byte6]
  [Byte8] -> Process GET_DAQ/8(Byte8)
  [Byte7] -> Process GET_DAQ/7(Byte7)
  [Byte6] -> Process GET_DAQ/6(Byte6)
  [Byte5] -> Process GET_DAQ/5(Byte5)
  [Byte4] -> Process GET_DAQ/4(Byte4)
  [Byte3] -> Process GET_DAQ/3(Byte3)
  [Byte2] -> Process GET_DAQ/2(Byte2)
  [Byte1] -> Process GET_DAQ/1(Byte1)
  [Byte8] -> Process WRITE_DAQ/8(Byte8)
  [Byte7] -> Process WRITE_DAQ/7(Byte7)
  [Byte6] -> Process WRITE_DAQ/6(Byte6)
  [Byte5] -> Process WRITE_DAQ/5(Byte5)
  [Byte4] -> Process WRITE_DAQ/4(Byte4)
  [Byte3] -> Process WRITE_DAQ/3(Byte3)
  [Byte2] -> Process WRITE_DAQ/2(Byte2)
  [Byte1] -> Process WRITE_DAQ/1(Byte1)
  Process WRITE_DAQ/1(CMD_info) -> WRITE/1
  CCP_Raw/1 -> Demux/1
  Process GET_DAQ/1(CMD_info) -> GET/1
  Process SET_DAQ/1(CMD_info) -> SET/1
  GET_DAQ/1 -> Relational Operator1/1
  SET_DAQ/1 -> Relational Operator3/1
  WRITE_DAQ/1 -> Relational Operator4/1
  [Byte1] -> Relational Operator3/2, Relational Operator4/2, Relational Operator1/2
  Logical Operator1/1 -> Switch1/2, Switch4/2

== system EmE_MBD_Blockset/User-Defined Functions/Snoop/CCP_ETC_SS1/Recieve Count ==
  Add : Sum  AccumDataTypeStr=uint8  OutDataTypeStr=uint8
  Constant : Constant  OutDataTypeStr=uint8
  Unit Delay : UnitDelay  SampleTime=-1
  motohawk_probe : MotoHawk_lib/Calibration & Probing Blocks/motohawk_probe  nam='CCP_Snoop_ATIcmd_cnt'  show_more=on  name_source=Use Parameter  read_level=1  view_as=Number  enum_struct={'Disabled', 'Enabled'}  vector_style=Wide Row  use_help_units=off  help=''  units=''  use_header_enum=off  row_header_enum={}  col_header_enum={}  use_min_max=off  min_val=-inf  max_val=inf  use_precision=off  precision=''  gain=1  offset=0  exp=1  use_mototune_group=on  mototune_group='CCP_Snoop'
      settings: SourceProductName=MotoHawk
  wires:
  Constant/1 -> Add/1
  Add/1 -> motohawk_probe/1, Unit Delay/1
  Unit Delay/1 -> Add/2

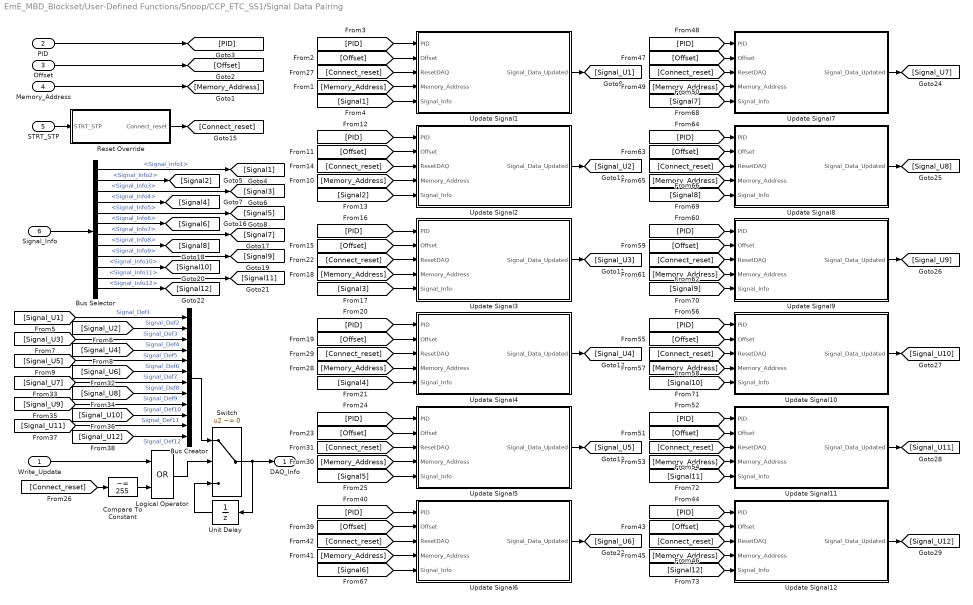
== system EmE_MBD_Blockset/User-Defined Functions/Snoop/CCP_ETC_SS1/Signal Data Pairing ==
  Write_Update : Inport
  PID : Inport  Port=2
  Offset : Inport  Port=3
  Memory_Address : Inport  Port=4
  STRT_STP : Inport  Port=5
  Signal_Info : Inport  Port=6
  Bus Creator : BusCreator  Inputs=12
  Bus Selector : BusSelector  OutputSignals=Signal_Info1,Signal_Info2,Signal_Info3,Signal_Info4,Signal_Info5,Signal_Info6,Signal_Info7,Signal_Info8,Signal_Info9,Signal_Info10,Signal_Info11,Signal_Info12
  Compare To Constant : simulink/Logic and Bit Operations/Compare To Constant  relop=~=  const=255  OutDataTypeStr=uint8
  Logical Operator : Logic  Operator=OR  AllPortsSameDT=off  OutDataTypeStr=boolean
  Reset Override : Subsystem
  Switch : Switch  Criteria=u2 ~= 0
  Unit Delay : UnitDelay  SampleTime=-1
  Update Signal1 : Subsystem
  Update Signal10 : Subsystem
  Update Signal11 : Subsystem
  Update Signal12 : Subsystem
  Update Signal2 : Subsystem
  Update Signal3 : Subsystem
  Update Signal4 : Subsystem
  Update Signal5 : Subsystem
  Update Signal6 : Subsystem
  Update Signal7 : Subsystem
  Update Signal8 : Subsystem
  Update Signal9 : Subsystem
  DAQ_Info : Outport
  wires:
  [Connect_reset] -> Compare To Constant/1
  Compare To Constant/1 -> Logical Operator/2
  Logical Operator/1 -> Switch/2
  [Signal6] -> Update Signal6/5(Signal_Info)
  [Signal7] -> Update Signal7/5(Signal_Info)
  [Signal8] -> Update Signal8/5(Signal_Info)
  [Signal9] -> Update Signal9/5(Signal_Info)
  [Signal10] -> Update Signal10/5(Signal_Info)
  [Signal11] -> Update Signal11/5(Signal_Info)
  [Signal12] -> Update Signal12/5(Signal_Info)
  Update Signal8/1(Signal_Data_Updated) -> [Signal_U8]
  Update Signal9/1(Signal_Data_Updated) -> [Signal_U9]
  Update Signal10/1(Signal_Data_Updated) -> [Signal_U10]
  Update Signal11/1(Signal_Data_Updated) -> [Signal_U11]
  Update Signal12/1(Signal_Data_Updated) -> [Signal_U12]
  Update Signal7/1(Signal_Data_Updated) -> [Signal_U7]
  Update Signal6/1(Signal_Data_Updated) -> [Signal_U6]
  [Memory_Address] -> Update Signal8/4(Memory_Address)
  [Connect_reset] -> Update Signal8/3(ResetDAQ)
  [Offset] -> Update Signal8/2(Offset)
  [PID] -> Update Signal8/1(PID)
  [Memory_Address] -> Update Signal9/4(Memory_Address)
  [Connect_reset] -> Update Signal9/3(ResetDAQ)
  [Offset] -> Update Signal9/2(Offset)
  [PID] -> Update Signal9/1(PID)
  [Memory_Address] -> Update Signal10/4(Memory_Address)
  [Connect_reset] -> Update Signal10/3(ResetDAQ)
  [Offset] -> Update Signal10/2(Offset)
  [PID] -> Update Signal10/1(PID)
  [Memory_Address] -> Update Signal11/4(Memory_Address)
  [Connect_reset] -> Update Signal11/3(ResetDAQ)
  [Offset] -> Update Signal11/2(Offset)
  [PID] -> Update Signal11/1(PID)
  [Memory_Address] -> Update Signal12/4(Memory_Address)
  [Connect_reset] -> Update Signal12/3(ResetDAQ)
  [Offset] -> Update Signal12/2(Offset)
  [PID] -> Update Signal12/1(PID)
  [Memory_Address] -> Update Signal7/4(Memory_Address)
  [Connect_reset] -> Update Signal7/3(ResetDAQ)
  [Offset] -> Update Signal7/2(Offset)
  [PID] -> Update Signal7/1(PID)
  [Memory_Address] -> Update Signal6/4(Memory_Address)
  [Connect_reset] -> Update Signal6/3(ResetDAQ)
  [Offset] -> Update Signal6/2(Offset)
  [PID] -> Update Signal6/1(PID)
  [Signal_U12] -> Bus Creator/12  "Signal_Def12"
  [Signal_U11] -> Bus Creator/11  "Signal_Def11"
  [Signal_U10] -> Bus Creator/10  "Signal_Def10"
  [Signal_U9] -> Bus Creator/9  "Signal_Def9"
  [Signal_U8] -> Bus Creator/8  "Signal_Def8"
  [Signal_U7] -> Bus Creator/7  "Signal_Def7"
  [Signal_U6] -> Bus Creator/6  "Signal_Def6"
  Bus Selector/12 -> [Signal12]  "<Signal_Info12>"
  Bus Selector/11 -> [Signal11]  "<Signal_Info11>"
  Bus Selector/10 -> [Signal10]  "<Signal_Info10>"
  Bus Selector/9 -> [Signal9]  "<Signal_Info9>"
  Bus Selector/8 -> [Signal8]  "<Signal_Info8>"
  Bus Selector/7 -> [Signal7]  "<Signal_Info7>"
  Bus Selector/6 -> [Signal6]  "<Signal_Info6>"
  [Memory_Address] -> Update Signal1/4(Memory_Address)
  [Connect_reset] -> Update Signal1/3(ResetDAQ)
  Reset Override/1(Connect_reset) -> [Connect_reset]
  STRT_STP/1 -> Reset Override/1(STRT_STP)
  [Signal5] -> Update Signal5/5(Signal_Info)
  [Memory_Address] -> Update Signal5/4(Memory_Address)
  [Connect_reset] -> Update Signal5/3(ResetDAQ)
  [Offset] -> Update Signal5/2(Offset)
  [PID] -> Update Signal5/1(PID)
  [Signal4] -> Update Signal4/5(Signal_Info)
  [Memory_Address] -> Update Signal4/4(Memory_Address)
  [Connect_reset] -> Update Signal4/3(ResetDAQ)
  [Offset] -> Update Signal4/2(Offset)
  [PID] -> Update Signal4/1(PID)
  [Signal3] -> Update Signal3/5(Signal_Info)
  [Memory_Address] -> Update Signal3/4(Memory_Address)
  [Connect_reset] -> Update Signal3/3(ResetDAQ)
  [Offset] -> Update Signal3/2(Offset)
  [PID] -> Update Signal3/1(PID)
  [Signal2] -> Update Signal2/5(Signal_Info)
  [Memory_Address] -> Update Signal2/4(Memory_Address)
  [Connect_reset] -> Update Signal2/3(ResetDAQ)
  [Offset] -> Update Signal2/2(Offset)
  [PID] -> Update Signal2/1(PID)
  [PID] -> Update Signal1/1(PID)
  [Offset] -> Update Signal1/2(Offset)
  [Signal1] -> Update Signal1/5(Signal_Info)
  Unit Delay/1 -> Switch/3
  Switch/1 -> Unit Delay/1, DAQ_Info/1
  Write_Update/1 -> Logical Operator/1
  Update Signal5/1(Signal_Data_Updated) -> [Signal_U5]
  Update Signal4/1(Signal_Data_Updated) -> [Signal_U4]
  Update Signal3/1(Signal_Data_Updated) -> [Signal_U3]
  Update Signal2/1(Signal_Data_Updated) -> [Signal_U2]
  [Signal_U1] -> Bus Creator/1  "Signal_Def1"
  [Signal_U2] -> Bus Creator/2  "Signal_Def2"
  [Signal_U3] -> Bus Creator/3  "Signal_Def3"
  [Signal_U4] -> Bus Creator/4  "Signal_Def4"
  [Signal_U5] -> Bus Creator/5  "Signal_Def5"
  Update Signal1/1(Signal_Data_Updated) -> [Signal_U1]
  Bus Selector/5 -> [Signal5]  "<Signal_Info5>"
  Bus Selector/4 -> [Signal4]  "<Signal_Info4>"
  Bus Selector/3 -> [Signal3]  "<Signal_Info3>"
  Bus Selector/2 -> [Signal2]  "<Signal_Info2>"
  Offset/1 -> [Offset]
  PID/1 -> [PID]
  Bus Selector/1 -> [Signal1]  "<Signal_Info1>"
  Signal_Info/1 -> Bus Selector/1
  Bus Creator/1 -> Switch/1
  Memory_Address/1 -> [Memory_Address]

== system EmE_MBD_Blockset/User-Defined Functions/Snoop/CCP_ETC_SS1/Update Detect ==
  CTR : Inport
  Newest_Cmd : Inport  Port=2
  Logical Operator2 : Logic  AllPortsSameDT=off  OutDataTypeStr=boolean
  Logical Operator3 : Logic  AllPortsSameDT=off  OutDataTypeStr=boolean
  Relational Operator : RelationalOperator  Operator=~=  OutDataTypeStr=boolean  RndMeth=Nearest
  Relational Operator1 : RelationalOperator  Operator===  OutDataTypeStr=boolean  RndMeth=Nearest
  Relational Operator3 : RelationalOperator  Operator===  OutDataTypeStr=boolean  RndMeth=Nearest
  SET_DAQ : Constant  Value=hex2dec('15')  OutDataTypeStr=uint8
  Unit Delay1 : UnitDelay  SampleTime=-1
  WRITE_DAQ : Constant  Value=hex2dec('16')  OutDataTypeStr=uint8
  Write_Update : Outport
  Set_Update : Outport  Port=2
  wires:
  Unit Delay1/1 -> Relational Operator/2
  CTR/1 -> Unit Delay1/1, Relational Operator/1
  SET_DAQ/1 -> Relational Operator3/1
  WRITE_DAQ/1 -> Relational Operator1/1
  Relational Operator3/1 -> Logical Operator2/1
  Relational Operator1/1 -> Logical Operator3/2
  Newest_Cmd/1 -> Relational Operator1/2, Relational Operator3/2
  Logical Operator2/1 -> Set_Update/1
  Logical Operator3/1 -> Write_Update/1
  Relational Operator/1 -> Logical Operator2/2, Logical Operator3/1

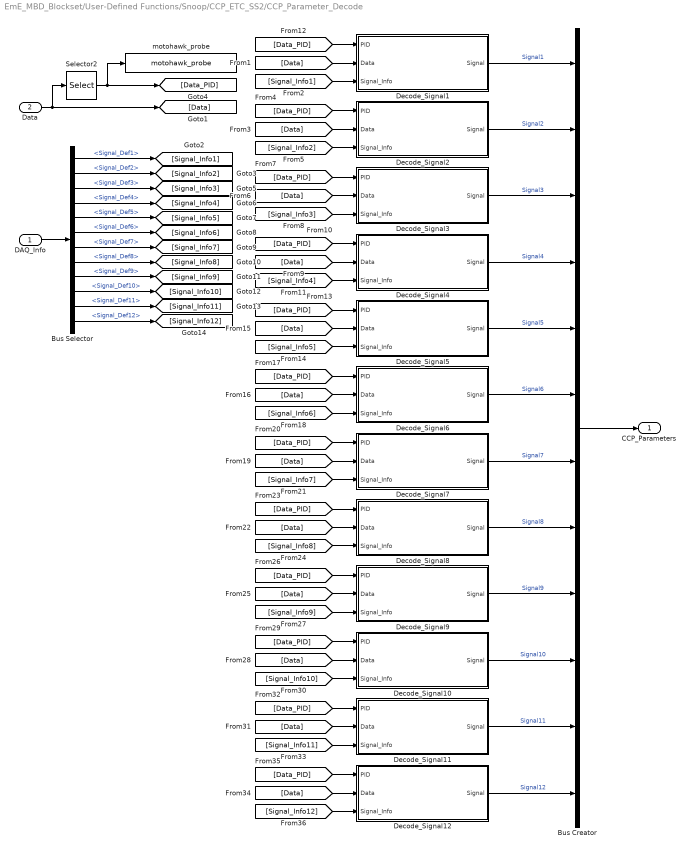
== system EmE_MBD_Blockset/User-Defined Functions/Snoop/CCP_ETC_SS2/CCP_Parameter_Decode ==
  DAQ_Info : Inport
  Data : Inport  Port=2
  Bus Creator : BusCreator  Inputs=12
  Bus Selector : BusSelector  OutputSignals=Signal_Def1,Signal_Def2,Signal_Def3,Signal_Def4,Signal_Def5,Signal_Def6,Signal_Def7,Signal_Def8,Signal_Def9,Signal_Def10,Signal_Def11,Signal_Def12
  Decode_Signal1 : Subsystem
  Decode_Signal10 : Subsystem
  Decode_Signal11 : Subsystem
  Decode_Signal12 : Subsystem
  Decode_Signal2 : Subsystem
  Decode_Signal3 : Subsystem
  Decode_Signal4 : Subsystem
  Decode_Signal5 : Subsystem
  Decode_Signal6 : Subsystem
  Decode_Signal7 : Subsystem
  Decode_Signal8 : Subsystem
  Decode_Signal9 : Subsystem
  Selector2 : Selector  InputPortWidth=8  IndexOptions=Index vector (dialog)  Indices=1  OutputSizes=1
  motohawk_probe : MotoHawk_lib/Calibration & Probing Blocks/motohawk_probe  nam='CCP_Snoop_CurrentPID'  show_more=on  name_source=Use Parameter  read_level=1  view_as=Number  enum_struct={'Disabled', 'Enabled'}  vector_style=Wide Row  use_help_units=off  help=''  units=''  use_header_enum=off  row_header_enum={}  col_header_enum={}  use_min_max=off  min_val=-inf  max_val=inf  use_precision=off  precision=''  gain=1  offset=0  exp=1  use_mototune_group=on  mototune_group='CCP_Snoop'
      settings: SourceProductName=MotoHawk
  CCP_Parameters : Outport
  wires:
  Decode_Signal12/1(Signal) -> Bus Creator/12  "Signal12"
  Decode_Signal11/1(Signal) -> Bus Creator/11  "Signal11"
  Decode_Signal10/1(Signal) -> Bus Creator/10  "Signal10"
  Decode_Signal9/1(Signal) -> Bus Creator/9  "Signal9"
  Decode_Signal8/1(Signal) -> Bus Creator/8  "Signal8"
  Decode_Signal7/1(Signal) -> Bus Creator/7  "Signal7"
  Decode_Signal6/1(Signal) -> Bus Creator/6  "Signal6"
  Decode_Signal5/1(Signal) -> Bus Creator/5  "Signal5"
  Decode_Signal4/1(Signal) -> Bus Creator/4  "Signal4"
  Decode_Signal3/1(Signal) -> Bus Creator/3  "Signal3"
  Decode_Signal2/1(Signal) -> Bus Creator/2  "Signal2"
  [Signal_Info6] -> Decode_Signal6/3(Signal_Info)
  [Data] -> Decode_Signal6/2(Data)
  [Data_PID] -> Decode_Signal6/1(PID)
  [Signal_Info7] -> Decode_Signal7/3(Signal_Info)
  [Data] -> Decode_Signal7/2(Data)
  [Data_PID] -> Decode_Signal7/1(PID)
  [Signal_Info8] -> Decode_Signal8/3(Signal_Info)
  [Data] -> Decode_Signal8/2(Data)
  [Data_PID] -> Decode_Signal8/1(PID)
  [Signal_Info9] -> Decode_Signal9/3(Signal_Info)
  [Data] -> Decode_Signal9/2(Data)
  [Data_PID] -> Decode_Signal9/1(PID)
  [Signal_Info10] -> Decode_Signal10/3(Signal_Info)
  [Data] -> Decode_Signal10/2(Data)
  [Data_PID] -> Decode_Signal10/1(PID)
  [Signal_Info11] -> Decode_Signal11/3(Signal_Info)
  [Data] -> Decode_Signal11/2(Data)
  [Data_PID] -> Decode_Signal11/1(PID)
  [Signal_Info12] -> Decode_Signal12/3(Signal_Info)
  [Data] -> Decode_Signal12/2(Data)
  [Data_PID] -> Decode_Signal12/1(PID)
  [Signal_Info5] -> Decode_Signal5/3(Signal_Info)
  [Data] -> Decode_Signal5/2(Data)
  [Data_PID] -> Decode_Signal5/1(PID)
  Bus Selector/12 -> [Signal_Info12]  "<Signal_Def12>"
  Bus Selector/11 -> [Signal_Info11]  "<Signal_Def11>"
  Bus Selector/10 -> [Signal_Info10]  "<Signal_Def10>"
  Bus Selector/9 -> [Signal_Info9]  "<Signal_Def9>"
  Bus Selector/8 -> [Signal_Info8]  "<Signal_Def8>"
  Bus Selector/7 -> [Signal_Info7]  "<Signal_Def7>"
  Bus Selector/6 -> [Signal_Info6]  "<Signal_Def6>"
  Decode_Signal1/1(Signal) -> Bus Creator/1  "Signal1"
  [Signal_Info4] -> Decode_Signal4/3(Signal_Info)
  [Data] -> Decode_Signal4/2(Data)
  [Data_PID] -> Decode_Signal4/1(PID)
  [Signal_Info3] -> Decode_Signal3/3(Signal_Info)
  [Data] -> Decode_Signal3/2(Data)
  [Data_PID] -> Decode_Signal3/1(PID)
  [Signal_Info2] -> Decode_Signal2/3(Signal_Info)
  [Data] -> Decode_Signal2/2(Data)
  [Data_PID] -> Decode_Signal2/1(PID)
  Bus Creator/1 -> CCP_Parameters/1
  Bus Selector/5 -> [Signal_Info5]  "<Signal_Def5>"
  Bus Selector/4 -> [Signal_Info4]  "<Signal_Def4>"
  Bus Selector/3 -> [Signal_Info3]  "<Signal_Def3>"
  Bus Selector/2 -> [Signal_Info2]  "<Signal_Def2>"
  Bus Selector/1 -> [Signal_Info1]  "<Signal_Def1>"
  DAQ_Info/1 -> Bus Selector/1
  [Signal_Info1] -> Decode_Signal1/3(Signal_Info)
  [Data] -> Decode_Signal1/2(Data)
  [Data_PID] -> Decode_Signal1/1(PID)
  Selector2/1 -> [Data_PID], motohawk_probe/1
  Data/1 -> [Data], Selector2/1
